simulink model "Topo_02_pcm"  (R2013a)
settings: Solver=ode45  StartTime=0.0  StopTime=10.0  RelTol=1e-6
undefined symbols (not defined in the file): magnitude
(part 1 of 2)
settings Model: Creator=Gau  LastModifiedBy=Gau

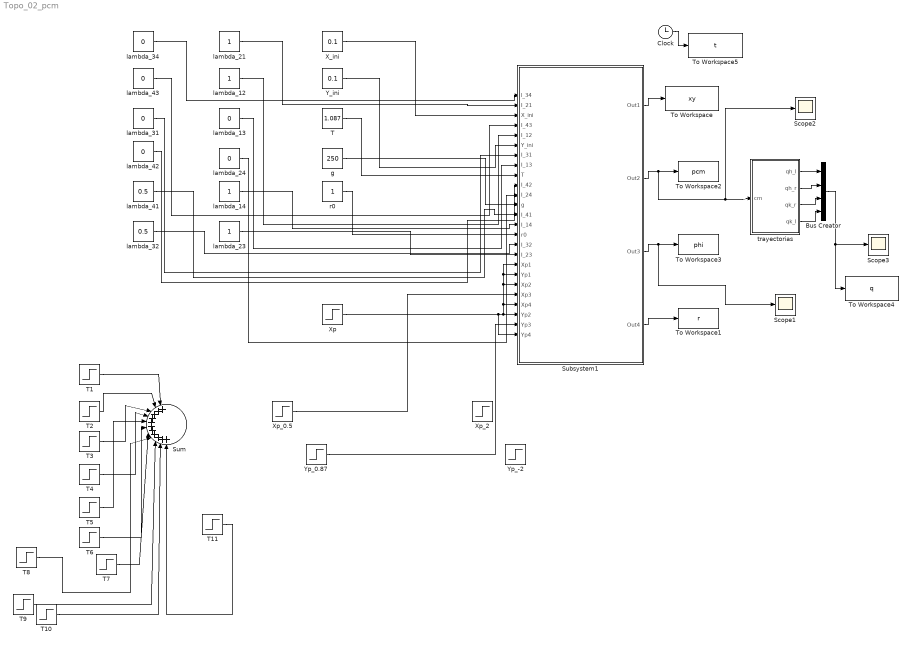
== system Topo_02_pcm ==
  Bus Creator : BusCreator
  Clock : Clock
  Scope1 : Scope
      settings: SaveName=ScopeData11
  Scope2 : Scope
      settings: SaveName=ScopeData2
  Scope3 : Scope
      settings: SaveName=ScopeData3
  Subsystem1 : Subsystem
  Sum : Sum  Inputs=|+++++++++++
  T : Constant  Value=1.087
  T1 : Step  Time=0  After=250  SampleTime=0
  T10 : Step  Time=9  After=50  SampleTime=0
  T11 : Step  Time=10  After=50  SampleTime=0
  T2 : Step  After=-240  SampleTime=0
  T3 : Step  Time=2  After=40  SampleTime=0
  T4 : Step  Time=3  After=50  SampleTime=0
  T5 : Step  Time=4  After=100  SampleTime=0
  T6 : Step  Time=5  After=100  SampleTime=0
  T7 : Step  Time=6  After=100  SampleTime=0
  T8 : Step  Time=7  After=50  SampleTime=0
  T9 : Step  Time=8  After=50  SampleTime=0
  To Workspace : ToWorkspace  VariableName=xy  SampleTime=-1
  To Workspace1 : ToWorkspace  VariableName=r  SampleTime=-1
  To Workspace2 : ToWorkspace  VariableName=pcm  SampleTime=-1
  To Workspace3 : ToWorkspace  VariableName=phi  SampleTime=-1
  To Workspace4 : ToWorkspace  VariableName=q  SampleTime=-1
  To Workspace5 : ToWorkspace  VariableName=t  SampleTime=-1
  X_ini : Constant  Value=0.1
  Xp : Step  Time=0  After=0  SampleTime=0
  Xp_0.5 : Step  Time=3  After=0.5  SampleTime=0
  Xp_2 : Step  Time=3  After=2  SampleTime=0
  Y_ini : Constant  Value=0.1
  Yp_-2 : Step  Time=3  After=-2  SampleTime=0
  Yp_0.87 : Step  Time=3  After=0.87  SampleTime=0
  g : Constant  Value=250
  lambda_{12,14,21,23} (4 alike) : Constant
  lambda_{13,24,34,42..43} (5 alike) : Constant  Value=0
  "lambda_31 " : Constant  Value=0
  lambda_32 : Constant  Value=0.5
  lambda_41 : Constant  Value=0.5
  r0 : Constant
  trayectorias : Subsystem
  wires:
  lambda_34/1 -> Subsystem1/1(l_34)
  lambda_21/1 -> Subsystem1/2(I_21)
  X_ini/1 -> Subsystem1/3(X_ini)
  lambda_43/1 -> Subsystem1/4(I_43)
  lambda_12/1 -> Subsystem1/5(I_12)
  Y_ini/1 -> Subsystem1/6(Y_ini)
  "lambda_31 "/1 -> Subsystem1/7(I_31)
  lambda_13/1 -> Subsystem1/8(I_13)
  lambda_42/1 -> Subsystem1/10(I_42)
  lambda_24/1 -> Subsystem1/11(I_24)
  g/1 -> Subsystem1/12(g)
  lambda_41/1 -> Subsystem1/13(I_41)
  lambda_14/1 -> Subsystem1/14(I_14)
  r0/1 -> Subsystem1/15(r0)
  lambda_32/1 -> Subsystem1/16(I_32)
  lambda_23/1 -> Subsystem1/17(I_23)
  Subsystem1/1(Out1) -> To Workspace/1
  Subsystem1/2(Out2) -> Scope2/1, trayectorias/1(cm), To Workspace2/1
  Subsystem1/3(Out3) -> Scope1/1, To Workspace3/1
  Subsystem1/4(Out4) -> To Workspace1/1
  trayectorias/1(qh_l) -> Bus Creator/1
  trayectorias/2(qh_r) -> Bus Creator/2
  trayectorias/3(qk_r) -> Bus Creator/3
  trayectorias/4(qk_l) -> Bus Creator/4
  Bus Creator/1 -> To Workspace4/1, Scope3/1
  Clock/1 -> To Workspace5/1
  T1/1 -> Sum/1
  T2/1 -> Sum/2
  T3/1 -> Sum/3
  T4/1 -> Sum/4
  T5/1 -> Sum/5
  T6/1 -> Sum/6
  T7/1 -> Sum/7
  T8/1 -> Sum/8
  T9/1 -> Sum/9
  T10/1 -> Sum/10
  T11/1 -> Sum/11
  T/1 -> Subsystem1/9(T)
  Xp/1 -> Subsystem1/23(Yp2), Subsystem1/22(Xp4), Subsystem1/20(Xp2), Subsystem1/18(Xp1), Subsystem1/19(Yp1), Subsystem1/25(Yp4)
  Xp_0.5/1 -> Subsystem1/21(Xp3)
  Yp_0.87/1 -> Subsystem1/24(Yp3)

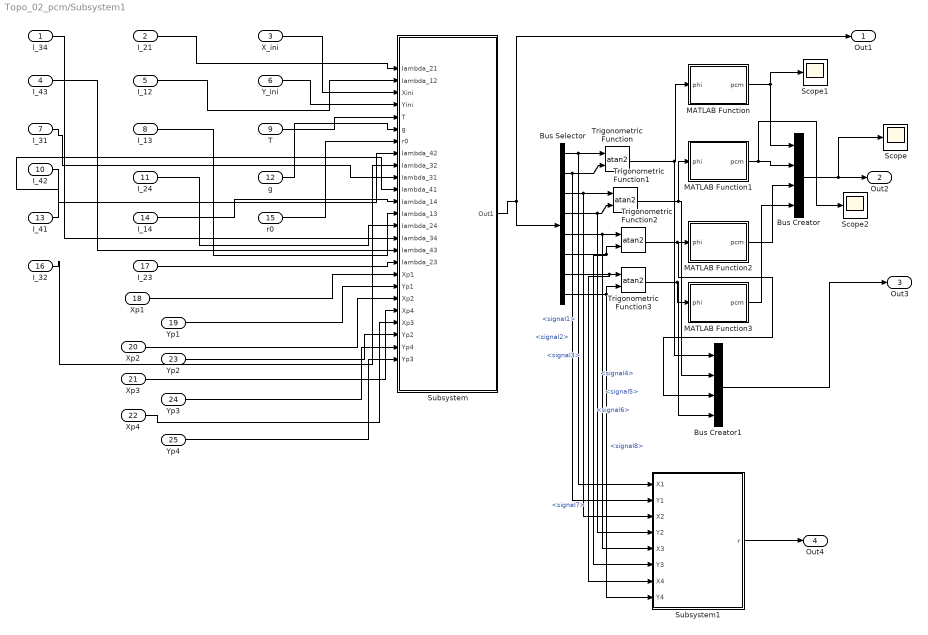
== system Topo_02_pcm/Subsystem1 ==
  l_34 : Inport
  I_21 : Inport  Port=2
  X_ini : Inport  Port=3
  I_43 : Inport  Port=4
  I_12 : Inport  Port=5
  Y_ini : Inport  Port=6
  I_31 : Inport  Port=7
  I_13 : Inport  Port=8
  T : Inport  Port=9
  I_42 : Inport  Port=10
  I_24 : Inport  Port=11
  g : Inport  Port=12
  I_41 : Inport  Port=13
  I_14 : Inport  Port=14
  r0 : Inport  Port=15
  I_32 : Inport  Port=16
  I_23 : Inport  Port=17
  Xp1 : Inport  Port=18
  Yp1 : Inport  Port=19
  Xp2 : Inport  Port=20
  Xp3 : Inport  Port=21
  Xp4 : Inport  Port=22
  Yp2 : Inport  Port=23
  Yp3 : Inport  Port=24
  Yp4 : Inport  Port=25
  Bus Creator : BusCreator
  Bus Creator1 : BusCreator
  Bus Selector : BusSelector  OutputSignals=signal1,signal2,signal3,signal4,signal5,signal6,signal7,signal8
  MATLAB Function : MATLAB Function  TreatAsAtomicUnit=on
  MATLAB Function1 : MATLAB Function  TreatAsAtomicUnit=on
  MATLAB Function2 : MATLAB Function  TreatAsAtomicUnit=on
  MATLAB Function3 : MATLAB Function  TreatAsAtomicUnit=on
  Scope : Scope
  Scope1 : Scope
      settings: TimeRange=10  SaveName=ScopeData9
  Scope2 : Scope
      settings: SaveName=ScopeData10
  Subsystem : Subsystem
  Subsystem1 : Subsystem
  Trigonometric Function{,1..3} (4 alike) : Trigonometry  Operator=atan2
  Out1 : Outport
  Out2 : Outport  Port=2
  Out3 : Outport  Port=3
  Out4 : Outport  Port=4
  wires:
  Trigonometric Function3/1 -> Bus Creator1/4, MATLAB Function3/1(phi)
  Bus Selector/7 -> Subsystem1/7(X4), Trigonometric Function3/1  "<signal7>"
  Bus Selector/8 -> Subsystem1/8(Y4), Trigonometric Function3/2  "<signal8>"
  Trigonometric Function1/1 -> Bus Creator1/2, MATLAB Function1/1(phi)
  Bus Selector/4 -> Subsystem1/4(Y2), Trigonometric Function1/2  "<signal4>"
  Trigonometric Function2/1 -> Bus Creator1/3, MATLAB Function2/1(phi)
  Bus Selector/5 -> Trigonometric Function2/1, Subsystem1/5(X3)  "<signal5>"
  Bus Selector/6 -> Trigonometric Function2/2, Subsystem1/6(Y3)  "<signal6>"
  Bus Selector/2 -> Subsystem1/2(Y1), Trigonometric Function/2  "<signal2>"
  Bus Creator/1 -> Scope/1, Out2/1
  Bus Creator1/1 -> Out3/1
  MATLAB Function/1(pcm) -> Bus Creator/1, Scope1/1
  MATLAB Function1/1(pcm) -> Scope2/1, Bus Creator/2
  MATLAB Function2/1(pcm) -> Bus Creator/3
  Subsystem/1(Out1) -> Bus Selector/1, Out1/1
  X_ini/1 -> Subsystem/3(Xini)
  Y_ini/1 -> Subsystem/4(Yini)
  T/1 -> Subsystem/5(T)
  g/1 -> Subsystem/6(g)
  r0/1 -> Subsystem/7(r0)
  I_21/1 -> Subsystem/1(Iambda_21)
  I_12/1 -> Subsystem/2(Iambda_12)
  I_42/1 -> Subsystem/8(Iambda_42)
  I_32/1 -> Subsystem/9(Iambda_32)
  I_31/1 -> Subsystem/10(lambda_31)
  I_41/1 -> Subsystem/11(lambda_41)
  I_14/1 -> Subsystem/12(Iambda_14)
  I_13/1 -> Subsystem/13(Iambda_13)
  I_24/1 -> Subsystem/14(Iambda_24)
  l_34/1 -> Subsystem/15(Iambda_34)
  I_43/1 -> Subsystem/16(Iambda_43)
  I_23/1 -> Subsystem/17(Iambda_23)
  Trigonometric Function/1 -> Bus Creator1/1, MATLAB Function/1(phi)
  Bus Selector/1 -> Subsystem1/1(X1), Trigonometric Function/1  "<signal1>"
  Bus Selector/3 -> Subsystem1/3(X2), Trigonometric Function1/1  "<signal3>"
  MATLAB Function3/1(pcm) -> Bus Creator/4
  Subsystem1/1(r) -> Out4/1
  Xp1/1 -> Subsystem/18(Xp1)
  Yp1/1 -> Subsystem/19(Yp1)
  Xp2/1 -> Subsystem/20(Xp2)
  Xp3/1 -> Subsystem/21(Xp4)
  Xp4/1 -> Subsystem/22(Xp3)
  Yp2/1 -> Subsystem/23(Yp2)
  Yp3/1 -> Subsystem/24(Yp4)
  Yp4/1 -> Subsystem/25(Yp3)

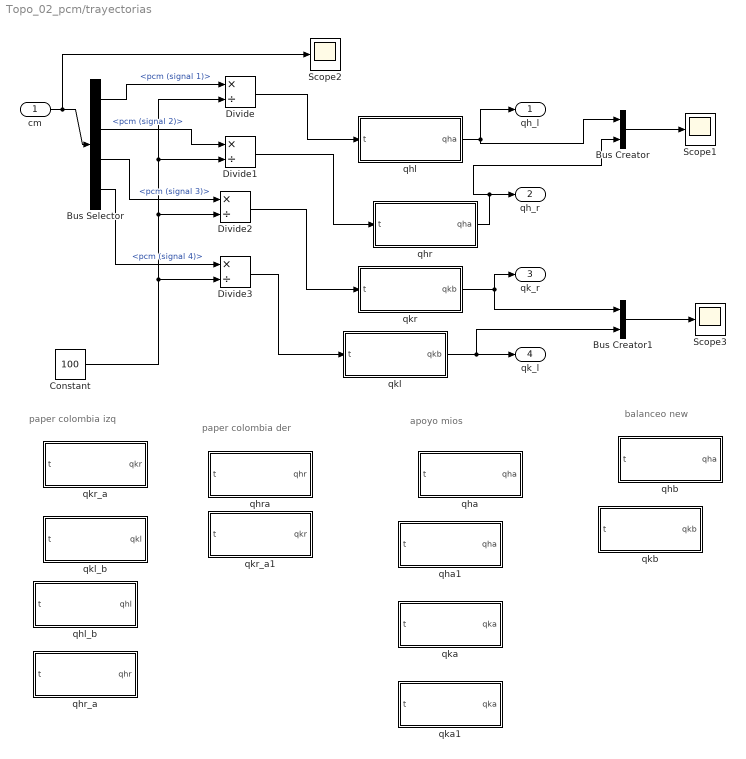
== system Topo_02_pcm/trayectorias ==
  note: balanceo new
  note: apoyo mios
  note: paper colombia der
  note: paper colombia izq
  cm : Inport
  Bus Creator : BusCreator  Inputs=2
  Bus Creator1 : BusCreator  Inputs=2
  Bus Selector : BusSelector  OutputSignals=pcm (signal 1),pcm (signal 2),pcm (signal 3),pcm (signal 4)
  Constant : Constant  Value=100
  Divide{,1..3} (4 alike) : Product  Inputs=*/
  Scope1 : Scope
  Scope2 : Scope
      settings: SaveName=ScopeData5
  Scope3 : Scope
      settings: SaveName=ScopeData4
  qha : Subsystem
  qha1 : Subsystem
  qhb : Subsystem
  qhl : Subsystem
  qhl_b : Subsystem
  qhr : Subsystem
  qhr_a : Subsystem
  qhra : Subsystem
  qka : Subsystem
  qka1 : Subsystem
  qkb : Subsystem
  qkl : Subsystem
  qkl_b : Subsystem
  qkr : Subsystem
  qkr_a : Subsystem
  qkr_a1 : Subsystem
  qh_l : Outport
  qh_r : Outport  Port=2
  qk_r : Outport  Port=3
  qk_l : Outport  Port=4
  wires:
  Constant/1 -> Divide3/2, Divide/2, Divide1/2, Divide2/2
  cm/1 -> Scope2/1, Bus Selector/1
  qkl/1(qkb) -> Bus Creator1/2, qk_l/1
  Divide3/1 -> qkl/1(t)
  Bus Selector/1 -> Divide/1  "<pcm (signal 1)>"
  Bus Selector/2 -> Divide1/1  "<pcm (signal 2)>"
  Bus Selector/3 -> Divide2/1  "<pcm (signal 3)>"
  Bus Selector/4 -> Divide3/1  "<pcm (signal 4)>"
  qhr/1(qha) -> Bus Creator/2, qh_r/1
  Divide1/1 -> qhr/1(t)
  Divide2/1 -> qkr/1(t)
  qkr/1(qkb) -> qk_r/1, Bus Creator1/1
  qhl/1(qha) -> Bus Creator/1, qh_l/1
  Bus Creator/1 -> Scope1/1
  Bus Creator1/1 -> Scope3/1
  Divide/1 -> qhl/1(t)

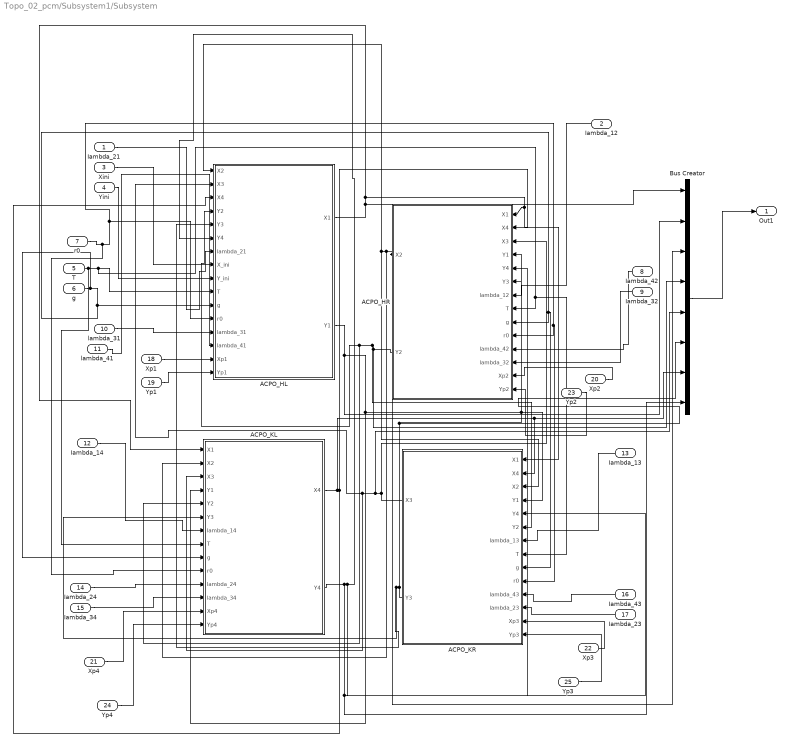
== system Topo_02_pcm/Subsystem1/Subsystem ==
  Iambda_21 : Inport
  Iambda_12 : Inport  Port=2
  Xini : Inport  Port=3
  Yini : Inport  Port=4
  T : Inport  Port=5
  g : Inport  Port=6
  r0 : Inport  Port=7
  Iambda_42 : Inport  Port=8
  Iambda_32 : Inport  Port=9
  lambda_31 : Inport  Port=10
  lambda_41 : Inport  Port=11
  Iambda_14 : Inport  Port=12
  Iambda_13 : Inport  Port=13
  Iambda_24 : Inport  Port=14
  Iambda_34 : Inport  Port=15
  Iambda_43 : Inport  Port=16
  Iambda_23 : Inport  Port=17
  Xp1 : Inport  Port=18
  Yp1 : Inport  Port=19
  Xp2 : Inport  Port=20
  Xp4 : Inport  Port=21
  Xp3 : Inport  Port=22
  Yp2 : Inport  Port=23
  Yp4 : Inport  Port=24
  Yp3 : Inport  Port=25
  ACPO_HL : Subsystem
  "ACPO_HR " : Subsystem
  ACPO_KL : Subsystem
  ACPO_KR : Subsystem
  Bus Creator : BusCreator  Inputs=8
  Out1 : Outport
  wires:
  ACPO_HL/2(Y1) -> Bus Creator/2, ACPO_KL/4(Y1), ACPO_KR/4(Y1), "ACPO_HR "/4(Y1)
  Iambda_21/1 -> ACPO_HL/7(lambda_21)
  Yini/1 -> ACPO_HL/9(Y_ini)
  g/1 -> ACPO_KL/9(g), "ACPO_HR "/9(g), ACPO_KR/9(g), ACPO_HL/11(g)
  r0/1 -> ACPO_KL/10(r0), "ACPO_HR "/10(r0), ACPO_KR/10(r0), ACPO_HL/12(r0)
  Iambda_24/1 -> ACPO_KL/11(lambda_24)
  Iambda_23/1 -> ACPO_KR/12(lambda_23)
  Iambda_13/1 -> ACPO_KR/7(lambda_13)
  ACPO_KL/2(Y4) -> Bus Creator/8, ACPO_KR/5(Y4), "ACPO_HR "/5(Y4), ACPO_HL/6(Y4)
  Xini/1 -> ACPO_HL/8(X_ini)
  Iambda_43/1 -> ACPO_KR/11(lambda_43)
  T/1 -> ACPO_KL/8(T), ACPO_KR/8(T), "ACPO_HR "/8(T), ACPO_HL/10(T)
  Iambda_14/1 -> ACPO_KL/7(lambda_14)
  lambda_41/1 -> ACPO_HL/14(lambda_41)
  Iambda_12/1 -> "ACPO_HR "/7(lambda_12)
  ACPO_HL/1(X1) -> ACPO_KL/1(X1), ACPO_KR/1(X1), "ACPO_HR "/1(X1), Bus Creator/1
  lambda_31/1 -> ACPO_HL/13(lambda_31)
  ACPO_KR/1(X3) -> Bus Creator/5, ACPO_HL/2(X3), ACPO_KL/3(X3), "ACPO_HR "/3(X3)
  Bus Creator/1 -> Out1/1
  Iambda_34/1 -> ACPO_KL/12(lambda_34)
  ACPO_KL/1(X4) -> Bus Creator/7, ACPO_KR/2(X4), "ACPO_HR "/2(X4), ACPO_HL/3(X4)
  Iambda_32/1 -> "ACPO_HR "/12(lambda_32)
  Iambda_42/1 -> "ACPO_HR "/11(lambda_42)
  "ACPO_HR "/2(Y2) -> ACPO_KR/6(Y2), ACPO_KL/5(Y2), ACPO_HL/4(Y2), Bus Creator/4
  "ACPO_HR "/1(X2) -> ACPO_KL/2(X2), ACPO_HL/1(X2), ACPO_KR/3(X2), Bus Creator/3
  ACPO_KR/2(Y3) -> "ACPO_HR "/6(Y3), Bus Creator/6, ACPO_KL/6(Y3), ACPO_HL/5(Y3)
  Xp1/1 -> ACPO_HL/15(Xp1)
  Yp1/1 -> ACPO_HL/16(Yp1)
  Xp2/1 -> "ACPO_HR "/13(Xp2)
  Xp4/1 -> ACPO_KL/13(Xp4)
  Xp3/1 -> ACPO_KR/13(Xp3)
  Yp2/1 -> "ACPO_HR "/14(Yp2)
  Yp4/1 -> ACPO_KL/14(Yp4)
  Yp3/1 -> ACPO_KR/14(Yp3)

== system Topo_02_pcm/Subsystem1/Subsystem1 ==
  X1 : Inport
  Y1 : Inport  Port=2
  X2 : Inport  Port=3
  Y2 : Inport  Port=4
  X3 : Inport  Port=5
  Y3 : Inport  Port=6
  X4 : Inport  Port=7
  Y4 : Inport  Port=8
  Add{,1..3} (4 alike) : Sum
  Bus Creator2 : BusCreator
  Fcn{,1..3} (4 alike) : Fcn  Expr=(1/sqrt(u))
  Product{,1..7} (8 alike) : Product
  r : Outport
  wires:
  Add/1 -> Fcn/1
  Product1/1 -> Add/2
  Product/1 -> Add/1
  Product2/1 -> Add1/1
  Product4/1 -> Add2/1
  Product6/1 -> Add3/1
  Product5/1 -> Add2/2
  Product3/1 -> Add1/2
  Add1/1 -> Fcn1/1
  Add3/1 -> Fcn3/1
  Add2/1 -> Fcn2/1
  Fcn3/1 -> Bus Creator2/4
  Product7/1 -> Add3/2
  Fcn2/1 -> Bus Creator2/3
  Fcn1/1 -> Bus Creator2/2
  Fcn/1 -> Bus Creator2/1
  Y4/1 -> Product7/2, Product7/1
  X4/1 -> Product6/1, Product6/2
  X2/1 -> Product2/2, Product2/1
  Y3/1 -> Product5/1, Product5/2
  X3/1 -> Product4/1, Product4/2
  Y2/1 -> Product3/2, Product3/1
  Bus Creator2/1 -> r/1
  Y1/1 -> Product1/2, Product1/1
  X1/1 -> Product/2, Product/1

== system Topo_02_pcm/trayectorias/qha ==
  t : Inport
  Add : Sum  Inputs=+++++++
  Constant : Constant  Value=14.3821853759039
  Divide{,1..3} (4 alike) : Product  Inputs=**
  Gain : Gain  Gain=-118.114739327716
  Gain1 : Gain  Gain=1234.01822080303
  Gain2 : Gain  Gain=-6454.06168266573
  Gain3 : Gain  Gain=13874.4402939381
  Gain4 : Gain  Gain=-12609.6480930329
  Gain5 : Gain  Gain=4065.04219370603
  Math Function : Math  Operator=magnitude^2  SaturateOnIntegerOverflow=on
  qha : Outport
  wires:
  t/1 -> Gain/1, Math Function/1, Divide/2, Divide1/2, Divide2/2, Divide3/2
  Math Function/1 -> Divide/1, Gain1/1
  Divide/1 -> Divide1/1, Gain2/1
  Divide1/1 -> Divide2/1, Gain3/1
  Divide2/1 -> Divide3/1, Gain4/1
  Divide3/1 -> Gain5/1
  Constant/1 -> Add/1
  Gain/1 -> Add/2
  Gain1/1 -> Add/3
  Gain2/1 -> Add/4
  Gain3/1 -> Add/5
  Gain4/1 -> Add/6
  Add/1 -> qha/1
  Gain5/1 -> Add/7

== system Topo_02_pcm/trayectorias/qha1 ==
  t : Inport
  Add : Sum  Inputs=+++++++
  Constant : Constant  Value=14.3821853759039
  Divide{,1..3} (4 alike) : Product  Inputs=**
  Gain : Gain  Gain=-118.114739327716
  Gain1 : Gain  Gain=1234.01822080303
  Gain2 : Gain  Gain=-6454.06168266573
  Gain3 : Gain  Gain=13874.4402939381
  Gain4 : Gain  Gain=-12609.6480930329
  Gain5 : Gain  Gain=4065.04219370603
  Math Function : Math  Operator=magnitude^2  SaturateOnIntegerOverflow=on
  qha : Outport
  wires:
  t/1 -> Gain/1, Math Function/1, Divide/2, Divide1/2, Divide2/2, Divide3/2
  Math Function/1 -> Divide/1, Gain1/1
  Divide/1 -> Divide1/1, Gain2/1
  Divide1/1 -> Divide2/1, Gain3/1
  Divide2/1 -> Divide3/1, Gain4/1
  Divide3/1 -> Gain5/1
  Constant/1 -> Add/1
  Gain/1 -> Add/2
  Gain1/1 -> Add/3
  Gain2/1 -> Add/4
  Gain3/1 -> Add/5
  Gain4/1 -> Add/6
  Add/1 -> qha/1
  Gain5/1 -> Add/7

== system Topo_02_pcm/trayectorias/qhb ==
  t : Inport
  Add : Sum  Inputs=++++++++
  Constant : Constant  Value=-3.7392
  Divide{,1..4} (5 alike) : Product  Inputs=**
  Gain : Gain  Gain=222.18
  Gain1 : Gain  Gain=370.54
  Gain2 : Gain  Gain=-8117.4
  Gain3 : Gain  Gain=27815
  Gain4 : Gain  Gain=-42622
  Gain5 : Gain  Gain=31114
  Gain6 : Gain  Gain=-8784.4
  Math Function : Math  Operator=magnitude^2  SaturateOnIntegerOverflow=on
  qha : Outport
  wires:
  t/1 -> Gain/1, Math Function/1, Divide/2, Divide1/2, Divide2/2, Divide4/2, Divide3/2
  Math Function/1 -> Divide/1, Gain1/1
  Divide/1 -> Divide1/1, Gain2/1
  Divide1/1 -> Divide2/1, Gain3/1
  Divide2/1 -> Divide3/1, Gain4/1
  Divide3/1 -> Divide4/1, Gain5/1
  Constant/1 -> Add/1
  Gain/1 -> Add/2
  Gain1/1 -> Add/3
  Gain2/1 -> Add/4
  Gain3/1 -> Add/5
  Gain4/1 -> Add/6
  Add/1 -> qha/1
  Gain5/1 -> Add/7
  Divide4/1 -> Gain6/1
  Gain6/1 -> Add/8

== system Topo_02_pcm/trayectorias/qhl ==
  t : Inport
  Add : Sum  Inputs=++++++++
  Constant : Constant  Value=-3.7392
  Divide{,1..4} (5 alike) : Product  Inputs=**
  Gain : Gain  Gain=222.18
  Gain1 : Gain  Gain=370.54
  Gain2 : Gain  Gain=-8117.4
  Gain3 : Gain  Gain=27815
  Gain4 : Gain  Gain=-42622
  Gain5 : Gain  Gain=31114
  Gain6 : Gain  Gain=-8784.4
  Math Function : Math  Operator=magnitude^2  SaturateOnIntegerOverflow=on
  qha : Outport
  wires:
  t/1 -> Gain/1, Math Function/1, Divide/2, Divide1/2, Divide2/2, Divide4/2, Divide3/2
  Math Function/1 -> Divide/1, Gain1/1
  Divide/1 -> Divide1/1, Gain2/1
  Divide1/1 -> Divide2/1, Gain3/1
  Divide2/1 -> Divide3/1, Gain4/1
  Divide3/1 -> Divide4/1, Gain5/1
  Constant/1 -> Add/1
  Gain/1 -> Add/2
  Gain1/1 -> Add/3
  Gain2/1 -> Add/4
  Gain3/1 -> Add/5
  Gain4/1 -> Add/6
  Add/1 -> qha/1
  Gain5/1 -> Add/7
  Divide4/1 -> Gain6/1
  Gain6/1 -> Add/8

== system Topo_02_pcm/trayectorias/qhl_b ==
  t : Inport
  Add : Sum  Inputs=+++++++
  Constant : Constant  Value=-4.6
  Divide{,1..3} (4 alike) : Product  Inputs=**
  Gain : Gain  Gain=-7
  Gain1 : Gain  Gain=1472.5
  Gain2 : Gain  Gain=-5330.8
  Gain3 : Gain  Gain=8017.4
  Gain4 : Gain  Gain=-5880.6
  Gain5 : Gain  Gain=1729
  Math Function : Math  Operator=magnitude^2  SaturateOnIntegerOverflow=on
  qhl : Outport
  wires:
  t/1 -> Gain/1, Math Function/1, Divide/2, Divide1/2, Divide2/2, Divide3/2
  Math Function/1 -> Divide/1, Gain1/1
  Divide/1 -> Divide1/1, Gain2/1
  Divide1/1 -> Divide2/1, Gain3/1
  Divide2/1 -> Divide3/1, Gain4/1
  Divide3/1 -> Gain5/1
  Constant/1 -> Add/1
  Gain/1 -> Add/2
  Gain1/1 -> Add/3
  Gain2/1 -> Add/4
  Gain3/1 -> Add/5
  Gain4/1 -> Add/6
  Add/1 -> qhl/1
  Gain5/1 -> Add/7

== system Topo_02_pcm/trayectorias/qhr ==
  t : Inport
  Add : Sum  Inputs=++++++++
  Constant : Constant  Value=-3.7392
  Divide{,1..4} (5 alike) : Product  Inputs=**
  Gain : Gain  Gain=222.18
  Gain1 : Gain  Gain=370.54
  Gain2 : Gain  Gain=-8117.4
  Gain3 : Gain  Gain=27815
  Gain4 : Gain  Gain=-42622
  Gain5 : Gain  Gain=31114
  Gain6 : Gain  Gain=-8784.4
  Math Function : Math  Operator=magnitude^2  SaturateOnIntegerOverflow=on
  qha : Outport
  wires:
  t/1 -> Gain/1, Math Function/1, Divide/2, Divide1/2, Divide2/2, Divide4/2, Divide3/2
  Math Function/1 -> Divide/1, Gain1/1
  Divide/1 -> Divide1/1, Gain2/1
  Divide1/1 -> Divide2/1, Gain3/1
  Divide2/1 -> Divide3/1, Gain4/1
  Divide3/1 -> Divide4/1, Gain5/1
  Constant/1 -> Add/1
  Gain/1 -> Add/2
  Gain1/1 -> Add/3
  Gain2/1 -> Add/4
  Gain3/1 -> Add/5
  Gain4/1 -> Add/6
  Add/1 -> qha/1
  Gain5/1 -> Add/7
  Divide4/1 -> Gain6/1
  Gain6/1 -> Add/8

== system Topo_02_pcm/trayectorias/qhr_a ==
  t : Inport
  Add : Sum  Inputs=+++++++
  Constant : Constant  Value=-4.6
  Divide{,1..3} (4 alike) : Product  Inputs=**
  Gain : Gain  Gain=-7
  Gain1 : Gain  Gain=1472.5
  Gain2 : Gain  Gain=-5330.8
  Gain3 : Gain  Gain=8017.4
  Gain4 : Gain  Gain=-5880.6
  Gain5 : Gain  Gain=1729
  Math Function : Math  Operator=magnitude^2  SaturateOnIntegerOverflow=on
  qhr : Outport
  wires:
  t/1 -> Gain/1, Math Function/1, Divide/2, Divide1/2, Divide2/2, Divide3/2
  Math Function/1 -> Divide/1, Gain1/1
  Divide/1 -> Divide1/1, Gain2/1
  Divide1/1 -> Divide2/1, Gain3/1
  Divide2/1 -> Divide3/1, Gain4/1
  Divide3/1 -> Gain5/1
  Constant/1 -> Add/1
  Gain/1 -> Add/2
  Gain1/1 -> Add/3
  Gain2/1 -> Add/4
  Gain3/1 -> Add/5
  Gain4/1 -> Add/6
  Add/1 -> qhr/1
  Gain5/1 -> Add/7

== system Topo_02_pcm/trayectorias/qhra ==
  t : Inport
  Add : Sum  Inputs=+++++++
  Constant : Constant  Value=39
  Divide{,1..3} (4 alike) : Product  Inputs=**
  Gain : Gain  Gain=-120
  Gain1 : Gain  Gain=1102
  Gain2 : Gain  Gain=-6967
  Gain3 : Gain  Gain=16201
  Gain4 : Gain  Gain=-15325
  Gain5 : Gain  Gain=5106
  Math Function : Math  Operator=magnitude^2  SaturateOnIntegerOverflow=on
  qhr : Outport
  wires:
  t/1 -> Gain/1, Math Function/1, Divide/2, Divide1/2, Divide2/2, Divide3/2
  Math Function/1 -> Divide/1, Gain1/1
  Divide/1 -> Divide1/1, Gain2/1
  Divide1/1 -> Divide2/1, Gain3/1
  Divide2/1 -> Divide3/1, Gain4/1
  Divide3/1 -> Gain5/1
  Constant/1 -> Add/1
  Gain/1 -> Add/2
  Gain1/1 -> Add/3
  Gain2/1 -> Add/4
  Gain3/1 -> Add/5
  Gain4/1 -> Add/6
  Add/1 -> qhr/1
  Gain5/1 -> Add/7

== system Topo_02_pcm/trayectorias/qka ==
  t : Inport
  Add : Sum  Inputs=+++++++
  Constant : Constant  Value=0.818814680699838
  Divide{,1..3} (4 alike) : Product  Inputs=**
  Gain : Gain  Gain=13.3308660372007
  Gain1 : Gain  Gain=2481.87072559977
  Gain2 : Gain  Gain=-18819.9542475597
  Gain3 : Gain  Gain=49702.4835857738
  Gain4 : Gain  Gain=-53863.1033124045
  Gain5 : Gain  Gain=20505.3942054591
  Math Function : Math  Operator=magnitude^2  SaturateOnIntegerOverflow=on
  qka : Outport
  wires:
  t/1 -> Gain/1, Math Function/1, Divide/2, Divide1/2, Divide2/2, Divide3/2
  Math Function/1 -> Divide/1, Gain1/1
  Divide/1 -> Divide1/1, Gain2/1
  Divide1/1 -> Divide2/1, Gain3/1
  Divide2/1 -> Divide3/1, Gain4/1
  Divide3/1 -> Gain5/1
  Constant/1 -> Add/1
  Gain/1 -> Add/2
  Gain1/1 -> Add/3
  Gain2/1 -> Add/4
  Gain3/1 -> Add/5
  Gain4/1 -> Add/6
  Add/1 -> qka/1
  Gain5/1 -> Add/7

== system Topo_02_pcm/trayectorias/qka1 ==
  t : Inport
  Add : Sum  Inputs=+++++++
  Constant : Constant  Value=0.818814680699838
  Divide{,1..3} (4 alike) : Product  Inputs=**
  Gain : Gain  Gain=13.3308660372007
  Gain1 : Gain  Gain=2481.87072559977
  Gain2 : Gain  Gain=-18819.9542475597
  Gain3 : Gain  Gain=49702.4835857738
  Gain4 : Gain  Gain=-53863.1033124045
  Gain5 : Gain  Gain=20505.3942054591
  Math Function : Math  Operator=magnitude^2  SaturateOnIntegerOverflow=on
  qka : Outport
  wires:
  t/1 -> Gain/1, Math Function/1, Divide/2, Divide1/2, Divide2/2, Divide3/2
  Math Function/1 -> Divide/1, Gain1/1
  Divide/1 -> Divide1/1, Gain2/1
  Divide1/1 -> Divide2/1, Gain3/1
  Divide2/1 -> Divide3/1, Gain4/1
  Divide3/1 -> Gain5/1
  Constant/1 -> Add/1
  Gain/1 -> Add/2
  Gain1/1 -> Add/3
  Gain2/1 -> Add/4
  Gain3/1 -> Add/5
  Gain4/1 -> Add/6
  Add/1 -> qka/1
  Gain5/1 -> Add/7

== system Topo_02_pcm/trayectorias/qkb ==
  t : Inport
  Add : Sum  Inputs=++++++++
  Constant : Constant  Value=43.515
  Divide{,1..4} (5 alike) : Product  Inputs=**
  Gain : Gain  Gain=591.34
  Gain1 : Gain  Gain=-3255.5
  Gain2 : Gain  Gain=-6144.4
  Gain3 : Gain  Gain=59007
  Gain4 : Gain  Gain=-121930
  Gain5 : Gain  Gain=104110
  Gain6 : Gain  Gain=-32382
  Math Function : Math  Operator=magnitude^2  SaturateOnIntegerOverflow=on
  qkb : Outport
  wires:
  t/1 -> Gain/1, Math Function/1, Divide/2, Divide1/2, Divide2/2, Divide4/1, Divide3/2
  Math Function/1 -> Divide/1, Gain1/1
  Divide/1 -> Divide1/1, Gain2/1
  Divide1/1 -> Divide2/1, Gain3/1
  Divide2/1 -> Divide3/1, Gain4/1
  Divide3/1 -> Divide4/2, Gain5/1
  Constant/1 -> Add/1
  Gain/1 -> Add/2
  Gain1/1 -> Add/3
  Gain2/1 -> Add/4
  Gain3/1 -> Add/5
  Gain4/1 -> Add/6
  Add/1 -> qkb/1
  Gain5/1 -> Add/7
  Divide4/1 -> Gain6/1
  Gain6/1 -> Add/8

== system Topo_02_pcm/trayectorias/qkl ==
  t : Inport
  Add : Sum  Inputs=++++++++
  Constant : Constant  Value=43.515
  Divide{,1..4} (5 alike) : Product  Inputs=**
  Gain : Gain  Gain=591.34
  Gain1 : Gain  Gain=-3255.5
  Gain2 : Gain  Gain=-6144.4
  Gain3 : Gain  Gain=59007
  Gain4 : Gain  Gain=-121930
  Gain5 : Gain  Gain=104110
  Gain6 : Gain  Gain=-32382
  Math Function : Math  Operator=magnitude^2  SaturateOnIntegerOverflow=on
  qkb : Outport
  wires:
  t/1 -> Gain/1, Math Function/1, Divide/2, Divide1/2, Divide2/2, Divide4/1, Divide3/2
  Math Function/1 -> Divide/1, Gain1/1
  Divide/1 -> Divide1/1, Gain2/1
  Divide1/1 -> Divide2/1, Gain3/1
  Divide2/1 -> Divide3/1, Gain4/1
  Divide3/1 -> Divide4/2, Gain5/1
  Constant/1 -> Add/1
  Gain/1 -> Add/2
  Gain1/1 -> Add/3
  Gain2/1 -> Add/4
  Gain3/1 -> Add/5
  Gain4/1 -> Add/6
  Add/1 -> qkb/1
  Gain5/1 -> Add/7
  Divide4/1 -> Gain6/1
  Gain6/1 -> Add/8

== system Topo_02_pcm/trayectorias/qkl_b ==
  t : Inport
  Add : Sum  Inputs=+++++++
  Constant : Constant  Value=-11
  Divide{,1..3} (4 alike) : Product  Inputs=**
  Gain : Gain  Gain=-152
  Gain1 : Gain  Gain=-3724
  Gain2 : Gain  Gain=25659
  Gain3 : Gain  Gain=-58222
  Gain4 : Gain  Gain=55828
  Gain5 : Gain  Gain=-19403
  Math Function : Math  Operator=magnitude^2  SaturateOnIntegerOverflow=on
  qkl : Outport
  wires:
  t/1 -> Gain/1, Math Function/1, Divide/2, Divide1/2, Divide2/2, Divide3/2
  Math Function/1 -> Divide/1, Gain1/1
  Divide/1 -> Divide1/1, Gain2/1
  Divide1/1 -> Divide2/1, Gain3/1
  Divide2/1 -> Divide3/1, Gain4/1
  Divide3/1 -> Gain5/1
  Constant/1 -> Add/1
  Gain/1 -> Add/2
  Gain1/1 -> Add/3
  Gain2/1 -> Add/4
  Gain3/1 -> Add/5
  Gain4/1 -> Add/6
  Add/1 -> qkl/1
  Gain5/1 -> Add/7

== system Topo_02_pcm/trayectorias/qkr ==
  t : Inport
  Add : Sum  Inputs=++++++++
  Constant : Constant  Value=43.515
  Divide{,1..4} (5 alike) : Product  Inputs=**
  Gain : Gain  Gain=591.34
  Gain1 : Gain  Gain=-3255.5
  Gain2 : Gain  Gain=-6144.4
  Gain3 : Gain  Gain=59007
  Gain4 : Gain  Gain=-121930
  Gain5 : Gain  Gain=104110
  Gain6 : Gain  Gain=-32382
  Math Function : Math  Operator=magnitude^2  SaturateOnIntegerOverflow=on
  qkb : Outport
  wires:
  t/1 -> Gain/1, Math Function/1, Divide/2, Divide1/2, Divide2/2, Divide4/1, Divide3/2
  Math Function/1 -> Divide/1, Gain1/1
  Divide/1 -> Divide1/1, Gain2/1
  Divide1/1 -> Divide2/1, Gain3/1
  Divide2/1 -> Divide3/1, Gain4/1
  Divide3/1 -> Divide4/2, Gain5/1
  Constant/1 -> Add/1
  Gain/1 -> Add/2
  Gain1/1 -> Add/3
  Gain2/1 -> Add/4
  Gain3/1 -> Add/5
  Gain4/1 -> Add/6
  Add/1 -> qkb/1
  Gain5/1 -> Add/7
  Divide4/1 -> Gain6/1
  Gain6/1 -> Add/8

== system Topo_02_pcm/trayectorias/qkr_a ==
  t : Inport
  Add : Sum  Inputs=+++++++
  Constant : Constant  Value=-11
  Divide{,1..3} (4 alike) : Product  Inputs=**
  Gain : Gain  Gain=-152
  Gain1 : Gain  Gain=-3724
  Gain2 : Gain  Gain=25659
  Gain3 : Gain  Gain=-58222
  Gain4 : Gain  Gain=55828
  Gain5 : Gain  Gain=-19403
  Math Function : Math  Operator=magnitude^2  SaturateOnIntegerOverflow=on
  qkr : Outport
  wires:
  t/1 -> Gain/1, Math Function/1, Divide/2, Divide1/2, Divide2/2, Divide3/2
  Math Function/1 -> Divide/1, Gain1/1
  Divide/1 -> Divide1/1, Gain2/1
  Divide1/1 -> Divide2/1, Gain3/1
  Divide2/1 -> Divide3/1, Gain4/1
  Divide3/1 -> Gain5/1
  Constant/1 -> Add/1
  Gain/1 -> Add/2
  Gain1/1 -> Add/3
  Gain2/1 -> Add/4
  Gain3/1 -> Add/5
  Gain4/1 -> Add/6
  Add/1 -> qkr/1
  Gain5/1 -> Add/7

== system Topo_02_pcm/trayectorias/qkr_a1 ==
  t : Inport
  Add : Sum  Inputs=+++++++
  Constant : Constant  Value=-6
  Divide{,1..3} (4 alike) : Product  Inputs=**
  Gain : Gain  Gain=-48
  Gain1 : Gain  Gain=-2013
  Gain2 : Gain  Gain=16109
  Gain3 : Gain  Gain=-42073
  Gain4 : Gain  Gain=44498
  Gain5 : Gain  Gain=-16470
  Math Function : Math  Operator=magnitude^2  SaturateOnIntegerOverflow=on
  qkr : Outport
  wires:
  t/1 -> Gain/1, Math Function/1, Divide/2, Divide1/2, Divide2/2, Divide3/2
  Math Function/1 -> Divide/1, Gain1/1
  Divide/1 -> Divide1/1, Gain2/1
  Divide1/1 -> Divide2/1, Gain3/1
  Divide2/1 -> Divide3/1, Gain4/1
  Divide3/1 -> Gain5/1
  Constant/1 -> Add/1
  Gain/1 -> Add/2
  Gain1/1 -> Add/3
  Gain2/1 -> Add/4
  Gain3/1 -> Add/5
  Gain4/1 -> Add/6
  Add/1 -> qkr/1
  Gain5/1 -> Add/7

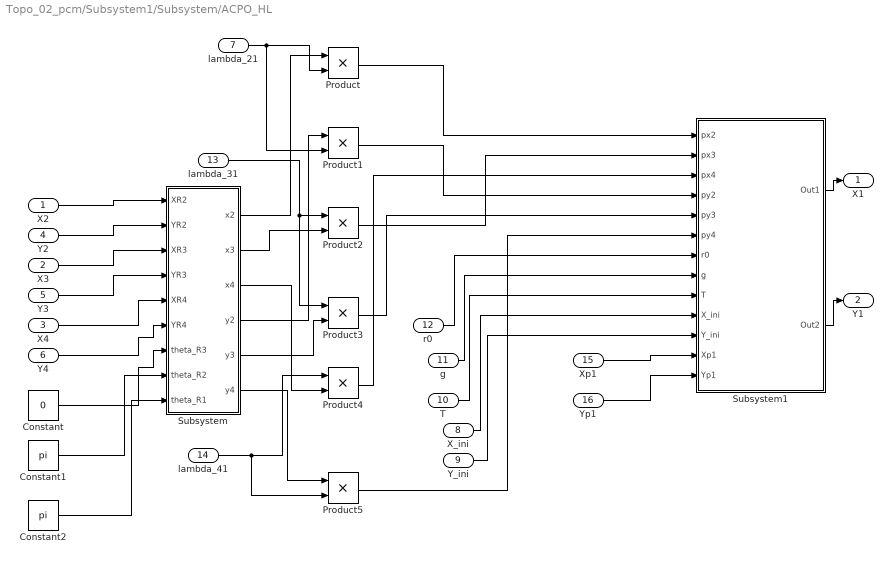
== system Topo_02_pcm/Subsystem1/Subsystem/ACPO_HL ==
  X2 : Inport
  X3 : Inport  Port=2
  X4 : Inport  Port=3
  Y2 : Inport  Port=4
  Y3 : Inport  Port=5
  Y4 : Inport  Port=6
  lambda_21 : Inport  Port=7
  X_ini : Inport  Port=8
  Y_ini : Inport  Port=9
  T : Inport  Port=10
  g : Inport  Port=11
  r0 : Inport  Port=12
  lambda_31 : Inport  Port=13
  lambda_41 : Inport  Port=14
  Xp1 : Inport  Port=15
  Yp1 : Inport  Port=16
  Constant : Constant  Value=0
  Constant1 : Constant  Value=pi
  Constant2 : Constant  Value=pi
  Product{,1..5} (6 alike) : Product
  Subsystem : Subsystem
  Subsystem1 : Subsystem
  X1 : Outport
  Y1 : Outport  Port=2
  wires:
  Subsystem1/1(Out1) -> X1/1
  Subsystem1/2(Out2) -> Y1/1
  X2/1 -> Subsystem/1(XR2)
  Y2/1 -> Subsystem/2(YR2)
  X3/1 -> Subsystem/3(XR3)
  Y3/1 -> Subsystem/4(YR3)
  X4/1 -> Subsystem/5(XR4)
  Y4/1 -> Subsystem/6(YR4)
  X_ini/1 -> Subsystem1/10(X_ini)
  Y_ini/1 -> Subsystem1/11(Y_ini)
  T/1 -> Subsystem1/9(T)
  g/1 -> Subsystem1/8(g)
  r0/1 -> Subsystem1/7(r0)
  Constant1/1 -> Subsystem/8(theta_R2)
  Constant2/1 -> Subsystem/9(theta_R1)
  Constant/1 -> Subsystem/7(theta_R3)
  Subsystem/1(x2) -> Product/1
  Subsystem/4(y2) -> Product1/1
  lambda_21/1 -> Product1/2, Product/2
  lambda_31/1 -> Product3/1, Product2/1
  Subsystem/2(x3) -> Product2/2
  Subsystem/5(y3) -> Product3/2
  Product/1 -> Subsystem1/1(px2)
  Product1/1 -> Subsystem1/4(py2)
  Product2/1 -> Subsystem1/2(px3)
  Product3/1 -> Subsystem1/5(py3)
  lambda_41/1 -> Product5/2, Product4/1
  Subsystem/3(x4) -> Product4/2
  Product4/1 -> Subsystem1/3(px4)
  Subsystem/6(y4) -> Product5/1
  Product5/1 -> Subsystem1/6(py4)
  Xp1/1 -> Subsystem1/12(Xp1)
  Yp1/1 -> Subsystem1/13(Yp1)

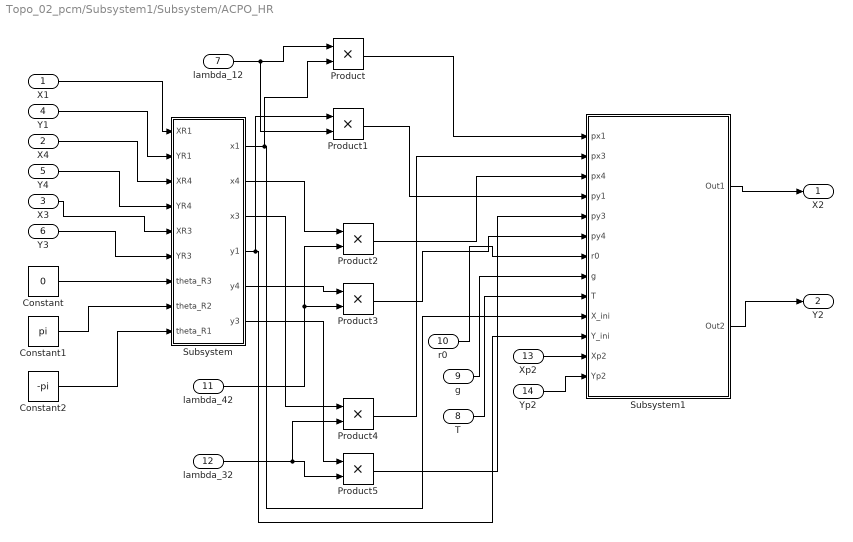
== system Topo_02_pcm/Subsystem1/Subsystem/ACPO_HR  ==
  X1 : Inport
  X4 : Inport  Port=2
  X3 : Inport  Port=3
  Y1 : Inport  Port=4
  Y4 : Inport  Port=5
  Y3 : Inport  Port=6
  lambda_12 : Inport  Port=7
  T : Inport  Port=8
  g : Inport  Port=9
  r0 : Inport  Port=10
  lambda_42 : Inport  Port=11
  lambda_32 : Inport  Port=12
  Xp2 : Inport  Port=13
  Yp2 : Inport  Port=14
  Constant : Constant  Value=0
  Constant1 : Constant  Value=pi
  Constant2 : Constant  Value=-pi
  Product{,1..5} (6 alike) : Product
  Subsystem : Subsystem
  Subsystem1 : Subsystem
  X2 : Outport
  Y2 : Outport  Port=2
  wires:
  Subsystem1/1(Out1) -> X2/1
  Subsystem1/2(Out2) -> Y2/1
  X1/1 -> Subsystem/1(XR1)
  Y1/1 -> Subsystem/2(YR1)
  X4/1 -> Subsystem/3(XR4)
  Y4/1 -> Subsystem/4(YR4)
  X3/1 -> Subsystem/5(XR3)
  Y3/1 -> Subsystem/6(YR3)
  T/1 -> Subsystem1/9(T)
  g/1 -> Subsystem1/8(g)
  r0/1 -> Subsystem1/7(r0)
  Constant1/1 -> Subsystem/8(theta_R2)
  Constant2/1 -> Subsystem/9(theta_R1)
  Constant/1 -> Subsystem/7(theta_R3)
  Subsystem/1(x1) -> Product/2, Subsystem1/10(X_ini)
  Subsystem/4(y1) -> Product1/1, Subsystem1/11(Y_ini)
  lambda_12/1 -> Product1/2, Product/1
  Product/1 -> Subsystem1/1(px1)
  Product1/1 -> Subsystem1/4(py1)
  lambda_42/1 -> Product3/2, Product2/2
  Subsystem/2(x4) -> Product2/1
  Product2/1 -> Subsystem1/3(px4)
  Subsystem/5(y4) -> Product3/1
  Product3/1 -> Subsystem1/6(py4)
  lambda_32/1 -> Product4/2, Product5/2
  Subsystem/3(x3) -> Product4/1
  Subsystem/6(y3) -> Product5/1
  Product4/1 -> Subsystem1/2(px3)
  Product5/1 -> Subsystem1/5(py3)
  Xp2/1 -> Subsystem1/12(Xp2)
  Yp2/1 -> Subsystem1/13(Yp2)

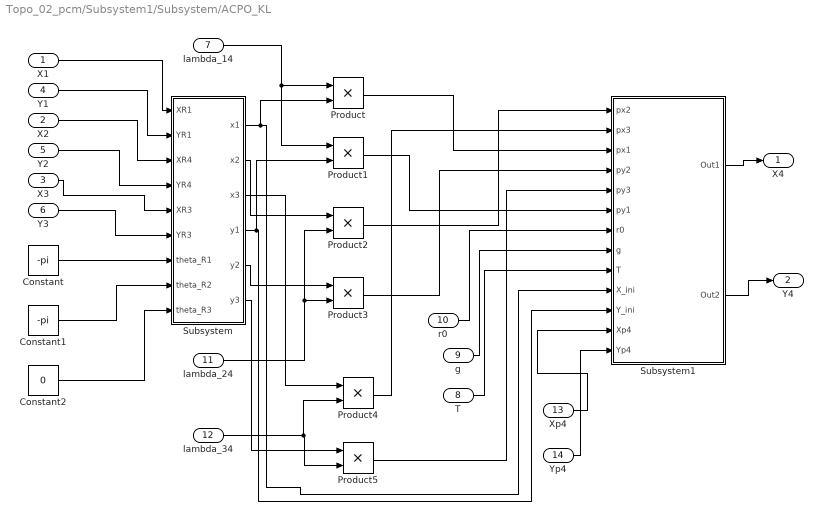
== system Topo_02_pcm/Subsystem1/Subsystem/ACPO_KL ==
  X1 : Inport
  X2 : Inport  Port=2
  X3 : Inport  Port=3
  Y1 : Inport  Port=4
  Y2 : Inport  Port=5
  Y3 : Inport  Port=6
  lambda_14 : Inport  Port=7
  T : Inport  Port=8
  g : Inport  Port=9
  r0 : Inport  Port=10
  lambda_24 : Inport  Port=11
  lambda_34 : Inport  Port=12
  Xp4 : Inport  Port=13
  Yp4 : Inport  Port=14
  Constant : Constant  Value=-pi
  Constant1 : Constant  Value=-pi
  Constant2 : Constant  Value=0
  Product{,1..5} (6 alike) : Product
  Subsystem : Subsystem
  Subsystem1 : Subsystem
  X4 : Outport
  Y4 : Outport  Port=2
  wires:
  Subsystem1/1(Out1) -> X4/1
  Subsystem1/2(Out2) -> Y4/1
  X1/1 -> Subsystem/1(XR1)
  Y1/1 -> Subsystem/2(YR1)
  X2/1 -> Subsystem/3(XR4)
  Y2/1 -> Subsystem/4(YR4)
  X3/1 -> Subsystem/5(XR3)
  Y3/1 -> Subsystem/6(YR3)
  T/1 -> Subsystem1/9(T)
  g/1 -> Subsystem1/8(g)
  r0/1 -> Subsystem1/7(r0)
  Constant1/1 -> Subsystem/8(theta_R2)
  Constant2/1 -> Subsystem/9(theta_R3)
  Constant/1 -> Subsystem/7(theta_R1)
  Subsystem/1(x1) -> Product/2, Subsystem1/10(X_ini)
  Subsystem/4(y1) -> Product1/2, Subsystem1/11(Y_ini)
  lambda_14/1 -> Product1/1, Product/1
  Product/1 -> Subsystem1/3(px1)
  Product1/1 -> Subsystem1/6(py1)
  lambda_24/1 -> Product3/2, Product2/2
  Subsystem/2(x2) -> Product2/1
  Subsystem/5(y2) -> Product3/1
  Product2/1 -> Subsystem1/1(px2)
  Product3/1 -> Subsystem1/4(py2)
  lambda_34/1 -> Product4/2, Product5/2
  Subsystem/3(x3) -> Product4/1
  Subsystem/6(y3) -> Product5/1
  Product4/1 -> Subsystem1/2(px3)
  Product5/1 -> Subsystem1/5(py3)
  Xp4/1 -> Subsystem1/12(Xp4)
  Yp4/1 -> Subsystem1/13(Yp4)

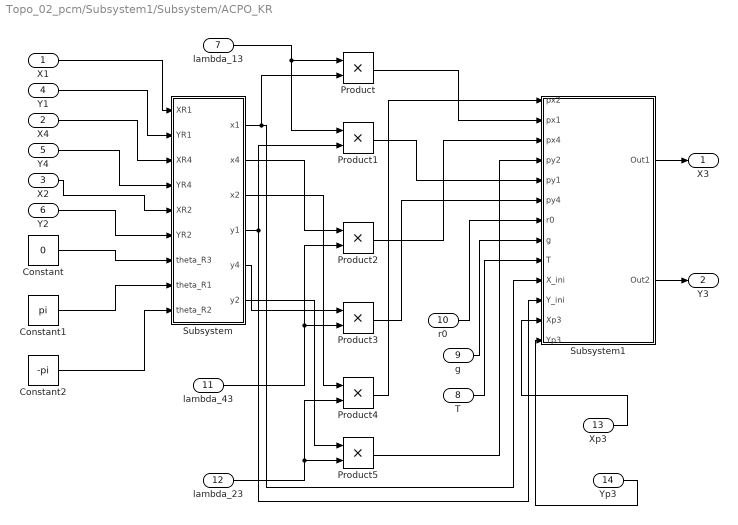
== system Topo_02_pcm/Subsystem1/Subsystem/ACPO_KR ==
  X1 : Inport
  X4 : Inport  Port=2
  X2 : Inport  Port=3
  Y1 : Inport  Port=4
  Y4 : Inport  Port=5
  Y2 : Inport  Port=6
  lambda_13 : Inport  Port=7
  T : Inport  Port=8
  g : Inport  Port=9
  r0 : Inport  Port=10
  lambda_43 : Inport  Port=11
  lambda_23 : Inport  Port=12
  Xp3 : Inport  Port=13
  Yp3 : Inport  Port=14
  Constant : Constant  Value=0
  Constant1 : Constant  Value=pi
  Constant2 : Constant  Value=-pi
  Product{,1..5} (6 alike) : Product
  Subsystem : Subsystem
  Subsystem1 : Subsystem
  X3 : Outport
  Y3 : Outport  Port=2
  wires:
  Subsystem1/1(Out1) -> X3/1
  Subsystem1/2(Out2) -> Y3/1
  X1/1 -> Subsystem/1(XR1)
  Y1/1 -> Subsystem/2(YR1)
  X4/1 -> Subsystem/3(XR4)
  Y4/1 -> Subsystem/4(YR4)
  X2/1 -> Subsystem/5(XR2)
  Y2/1 -> Subsystem/6(YR2)
  T/1 -> Subsystem1/9(T)
  g/1 -> Subsystem1/8(g)
  r0/1 -> Subsystem1/7(r0)
  Constant1/1 -> Subsystem/8(theta_R1)
  Constant2/1 -> Subsystem/9(theta_R2)
  Constant/1 -> Subsystem/7(theta_R3)
  Subsystem/1(x1) -> Product/2, Subsystem1/10(X_ini)
  Subsystem/4(y1) -> Subsystem1/11(Y_ini), Product1/2
  lambda_13/1 -> Product1/1, Product/1
  Product/1 -> Subsystem1/2(px1)
  Product1/1 -> Subsystem1/5(py1)
  lambda_43/1 -> Product3/2, Product2/2
  Subsystem/2(x4) -> Product2/1
  Subsystem/5(y4) -> Product3/1
  Product2/1 -> Subsystem1/3(px4)
  Product3/1 -> Subsystem1/6(py4)
  lambda_23/1 -> Product4/2, Product5/2
  Subsystem/3(x2) -> Product4/1
  Product4/1 -> Subsystem1/1(px2)
  Subsystem/6(y2) -> Product5/1
  Product5/1 -> Subsystem1/4(py2)
  Xp3/1 -> Subsystem1/12(Xp3)
  Yp3/1 -> Subsystem1/13(Yp3)

== system Topo_02_pcm/Subsystem1/Subsystem/ACPO_HL/Subsystem ==
  XR2 : Inport
  YR2 : Inport  Port=2
  XR3 : Inport  Port=3
  YR3 : Inport  Port=4
  XR4 : Inport  Port=5
  YR4 : Inport  Port=6
  theta_R3 : Inport  Port=7
  theta_R2 : Inport  Port=8
  theta_R1 : Inport  Port=9
  R1 : Subsystem
  R2 : Subsystem
  R3 : Subsystem
  x2 : Outport
  x3 : Outport  Port=2
  x4 : Outport  Port=3
  y2 : Outport  Port=4
  y3 : Outport  Port=5
  y4 : Outport  Port=6
  wires:
  XR2/1 -> R1/1(x)
  YR2/1 -> R1/2(y)
  R1/1(xr) -> x2/1
  R1/2(yr) -> y2/1
  XR3/1 -> R2/1(x)
  YR3/1 -> R2/2(y)
  theta_R2/1 -> R2/3(theta)
  R2/1(xr) -> x3/1
  R2/2(yr) -> y3/1
  XR4/1 -> R3/1(x)
  YR4/1 -> R3/2(y)
  theta_R3/1 -> R3/3(theta)
  R3/1(xr) -> x4/1
  R3/2(yr) -> y4/1
  theta_R1/1 -> R1/3(theta)

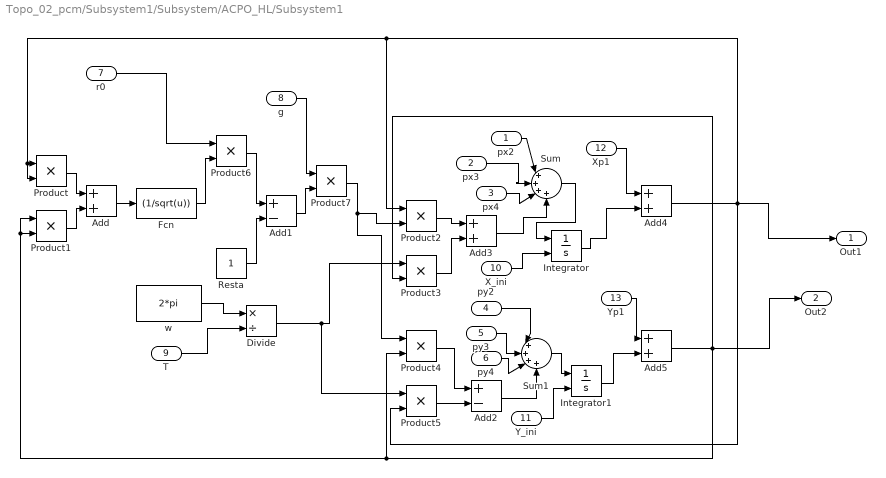
== system Topo_02_pcm/Subsystem1/Subsystem/ACPO_HL/Subsystem1 ==
  px2 : Inport
  px3 : Inport  Port=2
  px4 : Inport  Port=3
  py2 : Inport  Port=4
  py3 : Inport  Port=5
  py4 : Inport  Port=6
  r0 : Inport  Port=7
  g : Inport  Port=8
  T : Inport  Port=9
  X_ini : Inport  Port=10
  Y_ini : Inport  Port=11
  Xp1 : Inport  Port=12
  Yp1 : Inport  Port=13
  Add{,3..5} (4 alike) : Sum
  Add1 : Sum  Inputs=+-
  Add2 : Sum  Inputs=+-
  Divide : Product  Inputs=*/
  Fcn : Fcn  Expr=(1/sqrt(u))
  Integrator : Integrator  InitialConditionSource=external  InitialCondition=0.1
  Integrator1 : Integrator  InitialConditionSource=external  InitialCondition=0.1  IgnoreLimit=on
  Product{,1..7} (8 alike) : Product
  Resta : Constant  SampleTime=-1
  Sum : Sum  Inputs=|++++
  Sum1 : Sum  Inputs=|++++
  w : Constant  Value=2*pi  SampleTime=-1
  Out1 : Outport
  Out2 : Outport  Port=2
  wires:
  Add3/1 -> Sum/4
  Integrator/1 -> Add4/2
  Fcn/1 -> Product6/2
  r0/1 -> Product6/1
  w/1 -> Divide/1
  Product6/1 -> Add1/1
  T/1 -> Divide/2
  Divide/1 -> Product5/1, Product3/1
  Add2/1 -> Sum1/4
  Sum1/1 -> Integrator1/1
  Sum/1 -> Integrator/1
  Product4/1 -> Add2/1
  Product7/1 -> Product4/1, Product2/2
  Resta/1 -> Add1/2
  Add1/1 -> Product7/2
  Product3/1 -> Add3/2
  Integrator1/1 -> Add5/2
  Product5/1 -> Add2/2
  Product2/1 -> Add3/1
  Add/1 -> Fcn/1
  Product1/1 -> Add/2
  Product/1 -> Add/1
  py2/1 -> Sum1/1
  py4/1 -> Sum1/3
  py3/1 -> Sum1/2
  px2/1 -> Sum/1
  px4/1 -> Sum/3
  px3/1 -> Sum/2
  g/1 -> Product7/1
  X_ini/1 -> Integrator/2
  Y_ini/1 -> Integrator1/2
  Xp1/1 -> Add4/1
  Add4/1 -> Product5/2, Product2/1, Product/2, Product/1, Out1/1
  Add5/1 -> Out2/1, Product3/2, Product1/1, Product1/2, Product4/2
  Yp1/1 -> Add5/1

== system Topo_02_pcm/Subsystem1/Subsystem/ACPO_HR /Subsystem ==
  XR1 : Inport
  YR1 : Inport  Port=2
  XR4 : Inport  Port=3
  YR4 : Inport  Port=4
  XR3 : Inport  Port=5
  YR3 : Inport  Port=6
  theta_R3 : Inport  Port=7
  theta_R2 : Inport  Port=8
  theta_R1 : Inport  Port=9
  R1 : Subsystem
  R2 : Subsystem
  R3 : Subsystem
  x1 : Outport
  x4 : Outport  Port=2
  x3 : Outport  Port=3
  y1 : Outport  Port=4
  y4 : Outport  Port=5
  y3 : Outport  Port=6
  wires:
  XR1/1 -> R1/1(x)
  YR1/1 -> R1/2(y)
  R1/1(xr) -> x1/1
  R1/2(yr) -> y1/1
  XR4/1 -> R2/1(x)
  YR4/1 -> R2/2(y)
  theta_R2/1 -> R2/3(theta)
  R2/1(xr) -> x4/1
  R2/2(yr) -> y4/1
  XR3/1 -> R3/1(x)
  YR3/1 -> R3/2(y)
  theta_R3/1 -> R3/3(theta)
  R3/1(xr) -> x3/1
  R3/2(yr) -> y3/1
  theta_R1/1 -> R1/3(theta)

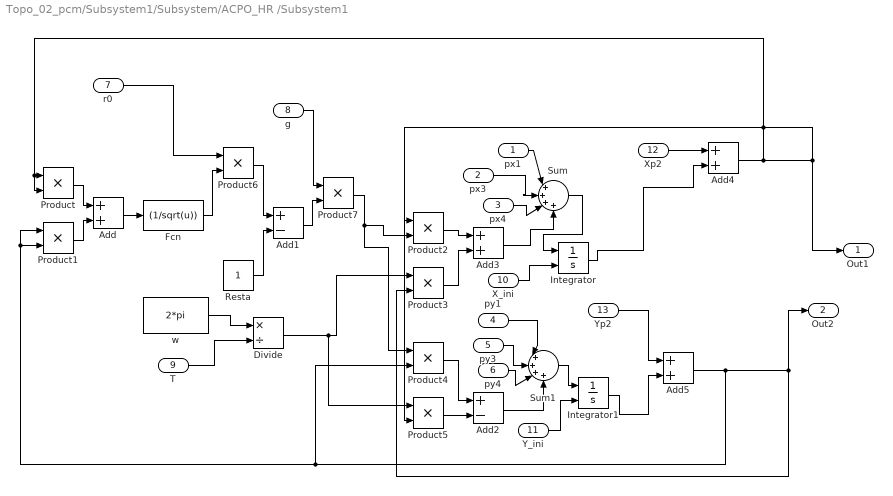
== system Topo_02_pcm/Subsystem1/Subsystem/ACPO_HR /Subsystem1 ==
  px1 : Inport
  px3 : Inport  Port=2
  px4 : Inport  Port=3
  py1 : Inport  Port=4
  py3 : Inport  Port=5
  py4 : Inport  Port=6
  r0 : Inport  Port=7
  g : Inport  Port=8
  T : Inport  Port=9
  X_ini : Inport  Port=10
  Y_ini : Inport  Port=11
  Xp2 : Inport  Port=12
  Yp2 : Inport  Port=13
  Add{,3..5} (4 alike) : Sum
  Add1 : Sum  Inputs=+-
  Add2 : Sum  Inputs=+-
  Divide : Product  Inputs=*/
  Fcn : Fcn  Expr=(1/sqrt(u))
  Integrator : Integrator  InitialConditionSource=external  InitialCondition=0.1
  Integrator1 : Integrator  InitialConditionSource=external  InitialCondition=0.1  IgnoreLimit=on
  Product{,1..7} (8 alike) : Product
  Resta : Constant  SampleTime=-1
  Sum : Sum  Inputs=|++++
  Sum1 : Sum  Inputs=|++++
  w : Constant  Value=2*pi  SampleTime=-1
  Out1 : Outport
  Out2 : Outport  Port=2
  wires:
  Add3/1 -> Sum/4
  Integrator/1 -> Add4/2
  Fcn/1 -> Product6/2
  r0/1 -> Product6/1
  w/1 -> Divide/1
  Product6/1 -> Add1/1
  T/1 -> Divide/2
  Divide/1 -> Product5/1, Product3/1
  Add2/1 -> Sum1/4
  Sum1/1 -> Integrator1/1
  Sum/1 -> Integrator/1
  Product4/1 -> Add2/1
  Product7/1 -> Product4/1, Product2/2
  Resta/1 -> Add1/2
  Add1/1 -> Product7/2
  Product3/1 -> Add3/2
  Integrator1/1 -> Add5/2
  Product5/1 -> Add2/2
  Product2/1 -> Add3/1
  Add/1 -> Fcn/1
  Product1/1 -> Add/2
  Product/1 -> Add/1
  py1/1 -> Sum1/1
  py4/1 -> Sum1/3
  py3/1 -> Sum1/2
  px1/1 -> Sum/1
  px4/1 -> Sum/3
  px3/1 -> Sum/2
  g/1 -> Product7/1
  X_ini/1 -> Integrator/2
  Y_ini/1 -> Integrator1/2
  Xp2/1 -> Add4/1
  Yp2/1 -> Add5/1
  Add4/1 -> Product2/1, Product/2, Product/1, Out1/1, Product5/2
  Add5/1 -> Product4/2, Product1/2, Product1/1, Product3/2, Out2/1

== system Topo_02_pcm/Subsystem1/Subsystem/ACPO_KL/Subsystem ==
  XR1 : Inport
  YR1 : Inport  Port=2
  XR4 : Inport  Port=3
  YR4 : Inport  Port=4
  XR3 : Inport  Port=5
  YR3 : Inport  Port=6
  theta_R1 : Inport  Port=7
  theta_R2 : Inport  Port=8
  theta_R3 : Inport  Port=9
  R1 : Subsystem
  R2 : Subsystem
  R3 : Subsystem
  x1 : Outport
  x2 : Outport  Port=2
  x3 : Outport  Port=3
  y1 : Outport  Port=4
  y2 : Outport  Port=5
  y3 : Outport  Port=6
  wires:
  XR1/1 -> R3/1(x)
  YR1/1 -> R3/2(y)
  R3/1(xr) -> x1/1
  R3/2(yr) -> y1/1
  XR4/1 -> R2/1(x)
  YR4/1 -> R2/2(y)
  theta_R2/1 -> R2/3(theta)
  R2/1(xr) -> x2/1
  R2/2(yr) -> y2/1
  XR3/1 -> R1/1(x)
  YR3/1 -> R1/2(y)
  theta_R1/1 -> R1/3(theta)
  R1/1(xr) -> x3/1
  R1/2(yr) -> y3/1
  theta_R3/1 -> R3/3(theta)

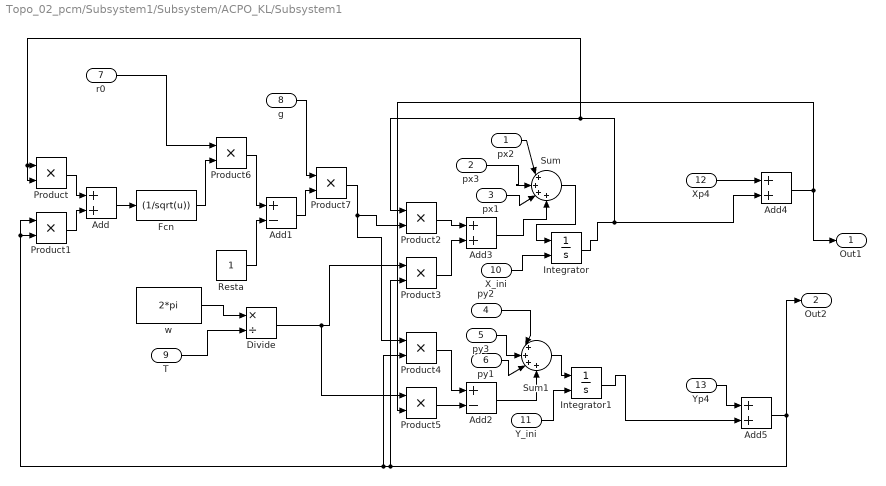
== system Topo_02_pcm/Subsystem1/Subsystem/ACPO_KL/Subsystem1 ==
  px2 : Inport
  px3 : Inport  Port=2
  px1 : Inport  Port=3
  py2 : Inport  Port=4
  py3 : Inport  Port=5
  py1 : Inport  Port=6
  r0 : Inport  Port=7
  g : Inport  Port=8
  T : Inport  Port=9
  X_ini : Inport  Port=10
  Y_ini : Inport  Port=11
  Xp4 : Inport  Port=12
  Yp4 : Inport  Port=13
  Add{,3..5} (4 alike) : Sum
  Add1 : Sum  Inputs=+-
  Add2 : Sum  Inputs=+-
  Divide : Product  Inputs=*/
  Fcn : Fcn  Expr=(1/sqrt(u))
  Integrator : Integrator  InitialConditionSource=external  InitialCondition=0.1
  Integrator1 : Integrator  InitialConditionSource=external  InitialCondition=0.1  IgnoreLimit=on
  Product{,1..7} (8 alike) : Product
  Resta : Constant  SampleTime=-1
  Sum : Sum  Inputs=|++++
  Sum1 : Sum  Inputs=|++++
  w : Constant  Value=2*pi  SampleTime=-1
  Out1 : Outport
  Out2 : Outport  Port=2
  wires:
  Add3/1 -> Sum/4
  Integrator/1 -> Product/2, Product/1, Product2/1, Add4/2
  Fcn/1 -> Product6/2
  r0/1 -> Product6/1
  w/1 -> Divide/1
  Product6/1 -> Add1/1
  T/1 -> Divide/2
  Divide/1 -> Product5/1, Product3/1
  Add2/1 -> Sum1/4
  Sum1/1 -> Integrator1/1
  Sum/1 -> Integrator/1
  Product4/1 -> Add2/1
  Product7/1 -> Product4/1, Product2/2
  Resta/1 -> Add1/2
  Add1/1 -> Product7/2
  Product3/1 -> Add3/2
  Integrator1/1 -> Add5/2
  Product5/1 -> Add2/2
  Product2/1 -> Add3/1
  Add/1 -> Fcn/1
  Product1/1 -> Add/2
  Product/1 -> Add/1
  py2/1 -> Sum1/1
  py1/1 -> Sum1/3
  py3/1 -> Sum1/2
  px2/1 -> Sum/1
  px1/1 -> Sum/3
  px3/1 -> Sum/2
  g/1 -> Product7/1
  X_ini/1 -> Integrator/2
  Y_ini/1 -> Integrator1/2
  Xp4/1 -> Add4/1
  Yp4/1 -> Add5/1
  Add4/1 -> Out1/1, Product5/2
  Add5/1 -> Out2/1, Product1/2, Product1/1, Product4/2, Product3/2

== system Topo_02_pcm/Subsystem1/Subsystem/ACPO_KR/Subsystem ==
  XR1 : Inport
  YR1 : Inport  Port=2
  XR4 : Inport  Port=3
  YR4 : Inport  Port=4
  XR2 : Inport  Port=5
  YR2 : Inport  Port=6
  theta_R3 : Inport  Port=7
  theta_R1 : Inport  Port=8
  theta_R2 : Inport  Port=9
  R1 : Subsystem
  R2 : Subsystem
  R3 : Subsystem
  x1 : Outport
  x4 : Outport  Port=2
  x2 : Outport  Port=3
  y1 : Outport  Port=4
  y4 : Outport  Port=5
  y2 : Outport  Port=6
  wires:
  XR1/1 -> R2/1(x)
  YR1/1 -> R2/2(y)
  R2/1(xr) -> x1/1
  R2/2(yr) -> y1/1
  XR4/1 -> R1/1(x)
  YR4/1 -> R1/2(y)
  theta_R1/1 -> R1/3(theta)
  R1/1(xr) -> x4/1
  R1/2(yr) -> y4/1
  XR2/1 -> R3/1(x)
  YR2/1 -> R3/2(y)
  theta_R3/1 -> R3/3(theta)
  R3/1(xr) -> x2/1
  R3/2(yr) -> y2/1
  theta_R2/1 -> R2/3(theta)

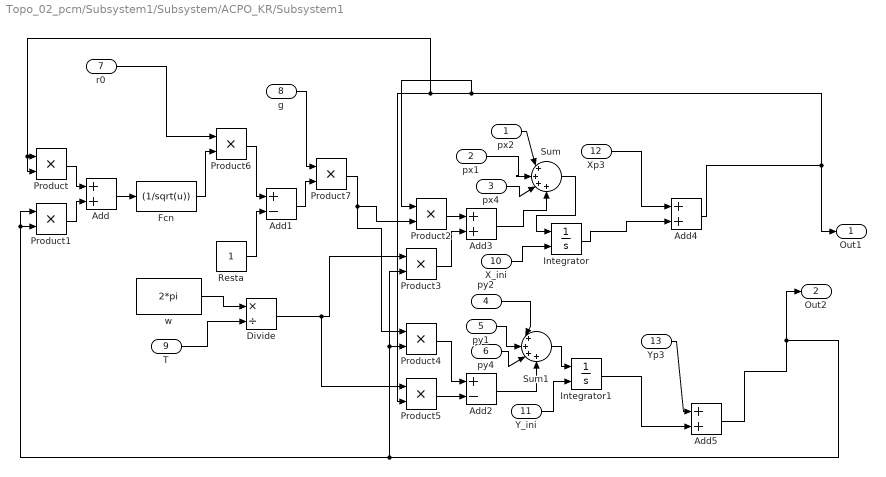
== system Topo_02_pcm/Subsystem1/Subsystem/ACPO_KR/Subsystem1 ==
  px2 : Inport
  px1 : Inport  Port=2
  px4 : Inport  Port=3
  py2 : Inport  Port=4
  py1 : Inport  Port=5
  py4 : Inport  Port=6
  r0 : Inport  Port=7
  g : Inport  Port=8
  T : Inport  Port=9
  X_ini : Inport  Port=10
  Y_ini : Inport  Port=11
  Xp3 : Inport  Port=12
  Yp3 : Inport  Port=13
  Add{,3..5} (4 alike) : Sum
  Add1 : Sum  Inputs=+-
  Add2 : Sum  Inputs=+-
  Divide : Product  Inputs=*/
  Fcn : Fcn  Expr=(1/sqrt(u))
  Integrator : Integrator  InitialConditionSource=external  InitialCondition=0.1
  Integrator1 : Integrator  InitialConditionSource=external  InitialCondition=0.1  IgnoreLimit=on
  Product{,1..7} (8 alike) : Product
  Resta : Constant  SampleTime=-1
  Sum : Sum  Inputs=|++++
  Sum1 : Sum  Inputs=|++++
  w : Constant  Value=2*pi  SampleTime=-1
  Out1 : Outport
  Out2 : Outport  Port=2
  wires:
  Add3/1 -> Sum/4
  Integrator/1 -> Add4/2
  Fcn/1 -> Product6/2
  r0/1 -> Product6/1
  w/1 -> Divide/1
  Product6/1 -> Add1/1
  T/1 -> Divide/2
  Divide/1 -> Product5/1, Product3/1
  Add2/1 -> Sum1/4
  Sum1/1 -> Integrator1/1
  Sum/1 -> Integrator/1
  Product4/1 -> Add2/1
  Product7/1 -> Product4/1, Product2/2
  Resta/1 -> Add1/2
  Add1/1 -> Product7/2
  Product3/1 -> Add3/2
  Product5/1 -> Add2/2
  Product2/1 -> Add3/1
  Add/1 -> Fcn/1
  Product1/1 -> Add/2
  Product/1 -> Add/1
  py2/1 -> Sum1/1
  py4/1 -> Sum1/3
  py1/1 -> Sum1/2
  px2/1 -> Sum/1
  px4/1 -> Sum/3
  px1/1 -> Sum/2
  g/1 -> Product7/1
  X_ini/1 -> Integrator/2
  Y_ini/1 -> Integrator1/2
  Xp3/1 -> Add4/1
  Yp3/1 -> Add5/1
  Add4/1 -> Out1/1, Product2/1, Product/2, Product/1, Product5/2
  Add5/1 -> Product1/2, Product1/1, Product4/2, Product3/2, Out2/1
  Integrator1/1 -> Add5/2

== system Topo_02_pcm/Subsystem1/Subsystem/ACPO_HL/Subsystem/R1 ==
  x : Inport
  y : Inport  Port=2
  theta : Inport  Port=3
  MATLAB Function1 : MATLAB Function  TreatAsAtomicUnit=on
  xr : Outport
  yr : Outport  Port=2
  wires:
  x/1 -> MATLAB Function1/1(x)
  y/1 -> MATLAB Function1/2(y)
  theta/1 -> MATLAB Function1/3(theta)
  MATLAB Function1/1(xr) -> xr/1
  MATLAB Function1/2(yr) -> yr/1

== system Topo_02_pcm/Subsystem1/Subsystem/ACPO_HL/Subsystem/R2 ==
  x : Inport
  y : Inport  Port=2
  theta : Inport  Port=3
  MATLAB Function1 : MATLAB Function  TreatAsAtomicUnit=on
  xr : Outport
  yr : Outport  Port=2
  wires:
  x/1 -> MATLAB Function1/1(x)
  y/1 -> MATLAB Function1/2(y)
  theta/1 -> MATLAB Function1/3(theta)
  MATLAB Function1/1(xr) -> xr/1
  MATLAB Function1/2(yr) -> yr/1

== system Topo_02_pcm/Subsystem1/Subsystem/ACPO_HL/Subsystem/R3 ==
  x : Inport
  y : Inport  Port=2
  theta : Inport  Port=3
  MATLAB Function1 : MATLAB Function  TreatAsAtomicUnit=on
  xr : Outport
  yr : Outport  Port=2
  wires:
  x/1 -> MATLAB Function1/1(x)
  y/1 -> MATLAB Function1/2(y)
  theta/1 -> MATLAB Function1/3(theta)
  MATLAB Function1/1(xr) -> xr/1
  MATLAB Function1/2(yr) -> yr/1

== system Topo_02_pcm/Subsystem1/Subsystem/ACPO_HR /Subsystem/R1 ==
  x : Inport
  y : Inport  Port=2
  theta : Inport  Port=3
  MATLAB Function1 : MATLAB Function  TreatAsAtomicUnit=on
  xr : Outport
  yr : Outport  Port=2
  wires:
  x/1 -> MATLAB Function1/1(x)
  y/1 -> MATLAB Function1/2(y)
  theta/1 -> MATLAB Function1/3(theta)
  MATLAB Function1/1(xr) -> xr/1
  MATLAB Function1/2(yr) -> yr/1

== system Topo_02_pcm/Subsystem1/Subsystem/ACPO_HR /Subsystem/R2 ==
  x : Inport
  y : Inport  Port=2
  theta : Inport  Port=3
  MATLAB Function1 : MATLAB Function  TreatAsAtomicUnit=on
  xr : Outport
  yr : Outport  Port=2
  wires:
  x/1 -> MATLAB Function1/1(x)
  y/1 -> MATLAB Function1/2(y)
  theta/1 -> MATLAB Function1/3(theta)
  MATLAB Function1/1(xr) -> xr/1
  MATLAB Function1/2(yr) -> yr/1

== system Topo_02_pcm/Subsystem1/Subsystem/ACPO_HR /Subsystem/R3 ==
  x : Inport
  y : Inport  Port=2
  theta : Inport  Port=3
  MATLAB Function1 : MATLAB Function  TreatAsAtomicUnit=on
  xr : Outport
  yr : Outport  Port=2
  wires:
  x/1 -> MATLAB Function1/1(x)
  y/1 -> MATLAB Function1/2(y)
  theta/1 -> MATLAB Function1/3(theta)
  MATLAB Function1/1(xr) -> xr/1
  MATLAB Function1/2(yr) -> yr/1

== system Topo_02_pcm/Subsystem1/Subsystem/ACPO_KL/Subsystem/R1 ==
  x : Inport
  y : Inport  Port=2
  theta : Inport  Port=3
  MATLAB Function1 : MATLAB Function  TreatAsAtomicUnit=on
  xr : Outport
  yr : Outport  Port=2
  wires:
  x/1 -> MATLAB Function1/1(x)
  y/1 -> MATLAB Function1/2(y)
  theta/1 -> MATLAB Function1/3(theta)
  MATLAB Function1/1(xr) -> xr/1
  MATLAB Function1/2(yr) -> yr/1

== system Topo_02_pcm/Subsystem1/Subsystem/ACPO_KL/Subsystem/R2 ==
  x : Inport
  y : Inport  Port=2
  theta : Inport  Port=3
  MATLAB Function1 : MATLAB Function  TreatAsAtomicUnit=on
  xr : Outport
  yr : Outport  Port=2
  wires:
  x/1 -> MATLAB Function1/1(x)
  y/1 -> MATLAB Function1/2(y)
  theta/1 -> MATLAB Function1/3(theta)
  MATLAB Function1/1(xr) -> xr/1
  MATLAB Function1/2(yr) -> yr/1

== system Topo_02_pcm/Subsystem1/Subsystem/ACPO_KL/Subsystem/R3 ==
  x : Inport
  y : Inport  Port=2
  theta : Inport  Port=3
  MATLAB Function1 : MATLAB Function  TreatAsAtomicUnit=on
  xr : Outport
  yr : Outport  Port=2
  wires:
  x/1 -> MATLAB Function1/1(x)
  y/1 -> MATLAB Function1/2(y)
  theta/1 -> MATLAB Function1/3(theta)
  MATLAB Function1/1(xr) -> xr/1
  MATLAB Function1/2(yr) -> yr/1

== system Topo_02_pcm/Subsystem1/Subsystem/ACPO_KR/Subsystem/R1 ==
  x : Inport
  y : Inport  Port=2
  theta : Inport  Port=3
  MATLAB Function1 : MATLAB Function  TreatAsAtomicUnit=on
  xr : Outport
  yr : Outport  Port=2
  wires:
  x/1 -> MATLAB Function1/1(x)
  y/1 -> MATLAB Function1/2(y)
  theta/1 -> MATLAB Function1/3(theta)
  MATLAB Function1/1(xr) -> xr/1
  MATLAB Function1/2(yr) -> yr/1

== system Topo_02_pcm/Subsystem1/Subsystem/ACPO_KR/Subsystem/R2 ==
  x : Inport
  y : Inport  Port=2
  theta : Inport  Port=3
  MATLAB Function1 : MATLAB Function  TreatAsAtomicUnit=on
  xr : Outport
  yr : Outport  Port=2
  wires:
  x/1 -> MATLAB Function1/1(x)
  y/1 -> MATLAB Function1/2(y)
  theta/1 -> MATLAB Function1/3(theta)
  MATLAB Function1/1(xr) -> xr/1
  MATLAB Function1/2(yr) -> yr/1

== system Topo_02_pcm/Subsystem1/Subsystem/ACPO_KR/Subsystem/R3 ==
  x : Inport
  y : Inport  Port=2
  theta : Inport  Port=3
  MATLAB Function1 : MATLAB Function  TreatAsAtomicUnit=on
  xr : Outport
  yr : Outport  Port=2
  wires:
  x/1 -> MATLAB Function1/1(x)
  y/1 -> MATLAB Function1/2(y)
  theta/1 -> MATLAB Function1/3(theta)
  MATLAB Function1/1(xr) -> xr/1
  MATLAB Function1/2(yr) -> yr/1

== matlab function Topo_02_pcm/Subsystem1/Subsystem/ACPO_HL/Subsystem/R1/MATLAB Function1 ==
  data: x input; y input; theta input; xr output; yr output
function [xr,yr]=Rot_theta(x,y,theta)
xr=[cos(theta) -sin(theta)]*[x y]';
yr=[sin(theta) cos(theta)]*[x y]';
end

== matlab function Topo_02_pcm/Subsystem1/MATLAB Function ==
  data: phi input; pcm output
function pcm=pcm(phi)
g=phi.*180./pi;
for i=1:length(g)
    if g(i)<0 
        g(i)=g(i)+360;
    end
end
pcm=g.*100./(360);

== matlab function Topo_02_pcm/Subsystem1/Subsystem/ACPO_HL/Subsystem/R2/MATLAB Function1 ==
  data: x input; y input; theta input; xr output; yr output
function [xr,yr]=Rot_theta(x,y,theta)
xr=[cos(theta) -sin(theta)]*[x y]';
yr=[sin(theta) cos(theta)]*[x y]';
end

== matlab function Topo_02_pcm/Subsystem1/Subsystem/ACPO_HL/Subsystem/R3/MATLAB Function1 ==
  data: x input; y input; theta input; xr output; yr output
function [xr,yr]=Rot_theta(x,y,theta)
xr=[cos(theta) -sin(theta)]*[x y]';
yr=[sin(theta) cos(theta)]*[x y]';
end

== matlab function Topo_02_pcm/Subsystem1/Subsystem/ACPO_HR /Subsystem/R1/MATLAB Function1 ==
  data: x input; y input; theta input; xr output; yr output
function [xr,yr]=Rot_theta(x,y,theta)
xr=[cos(theta) -sin(theta)]*[x y]';
yr=[sin(theta) cos(theta)]*[x y]';
end

== matlab function Topo_02_pcm/Subsystem1/Subsystem/ACPO_HR /Subsystem/R2/MATLAB Function1 ==
  data: x input; y input; theta input; xr output; yr output
function [xr,yr]=Rot_theta(x,y,theta)
xr=[cos(theta) -sin(theta)]*[x y]';
yr=[sin(theta) cos(theta)]*[x y]';
end

== matlab function Topo_02_pcm/Subsystem1/Subsystem/ACPO_HR /Subsystem/R3/MATLAB Function1 ==
  data: x input; y input; theta input; xr output; yr output
function [xr,yr]=Rot_theta(x,y,theta)
xr=[cos(theta) -sin(theta)]*[x y]';
yr=[sin(theta) cos(theta)]*[x y]';
end

== matlab function Topo_02_pcm/Subsystem1/Subsystem/ACPO_KR/Subsystem/R1/MATLAB Function1 ==
  data: x input; y input; theta input; xr output; yr output
function [xr,yr]=Rot_theta(x,y,theta)
xr=[cos(theta) -sin(theta)]*[x y]';
yr=[sin(theta) cos(theta)]*[x y]';
end

== matlab function Topo_02_pcm/Subsystem1/Subsystem/ACPO_KR/Subsystem/R2/MATLAB Function1 ==
  data: x input; y input; theta input; xr output; yr output
function [xr,yr]=Rot_theta(x,y,theta)
xr=[cos(theta) -sin(theta)]*[x y]';
yr=[sin(theta) cos(theta)]*[x y]';
end
